simulink model "emgCalibration"  (R2017a)
settings: Solver=ode5  StartTime=0.0  StopTime=10  FixedStep=Ts_sim  RelTol=1e-3  EnableMultiTasking=on
values from neighbouring files (symbols this model uses):
  emgConst2 = 0    [initializeParameters.m]
undefined symbols (not defined in the file or in its folder): A_butter_cal, A_butter_low, B_butter_cal, B_butter_low
libraries: robotlib x1
settings Model: Creator=Clark  LastModifiedBy=jacob
settings DataIOCC: LimitDataPoints=on  SaveFormat=Array
settings OptimizationCC: LifeSpan=inf
settings DebuggingCC: SFUnexpectedBacktrackingDiag=warning  SFNoUnconditionalDefaultTransitionDiag=warning  SFExecutionAtInitializationDiag=none
settings HardwareCC: ProdBitPerPointer=32  ProdBitPerSizeT=32  ProdBitPerPtrDiffT=32  ProdLargestAtomicFloat=None  ProdIntDivRoundTo=Undefined  ProdEndianess=Unspecified  ProdWordSize=32  ProdHWDeviceType=32-bit Generic
settings ModelReferenceCC: PropagateSignalLabelsOutOfModel=off
settings GRTTargetCC: TargetLangStandard=C89/C90 (ANSI)  GeneratePreprocessorConditionals=Disable all
settings ConfigComp: CovMetricSettings=dw  CovHtmlReporting=on  CovSaveCumulativeToWorkspaceVar=on  CovSaveSingleToWorkspaceVar=on  CovExternalEMLEnable=off

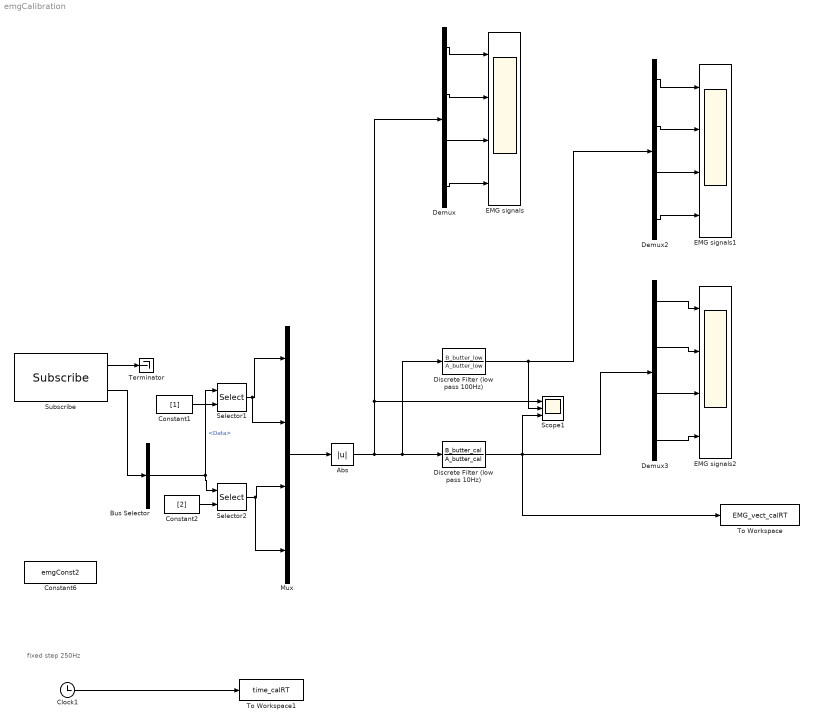
== system emgCalibration ==
  note: fixed step 250Hz
  Abs : Abs
  Bus Selector : BusSelector  OutputSignals=Data
  Clock1 : Clock
  Constant1 : Constant  Value=[1]
  Constant2 : Constant  Value=[2]
  Constant6 : Constant  Value=emgConst2  VectorParams1D=off  OutDataTypeStr=int16
  Demux : Demux
  Demux2 : Demux
  Demux3 : Demux
  Discrete Filter (low pass 100Hz) : DiscreteFilter  Numerator=B_butter_low  Denominator=A_butter_low
  Discrete Filter (low pass 10Hz) : DiscreteFilter  Numerator=B_butter_cal  Denominator=A_butter_cal
  EMG signals : Scope  NumInputPorts=4
  EMG signals1 : Scope  NumInputPorts=4
  EMG signals2 : Scope  NumInputPorts=4
  Mux : Mux
  Scope1 : Scope  NumInputPorts=3
  Selector1 : Selector  IndexOptions=Index vector (port)  Indices=[1 3]  OutputSizes=1
  Selector2 : Selector  IndexOptions=Index vector (port)  Indices=[1 3]  OutputSizes=1
  Subscribe : robotlib/Subscribe  SourceLibraryInfo=This block requires Robotics System Toolbox  topicSource=Select from ROS network  topic=/emgPub  messageType=std_msgs/Int16MultiArray  sampleTime=-1  messageQueueLength=1
      settings: SourceProductBaseCode=RO
  Terminator : Terminator
  To Workspace : ToWorkspace  VariableName=EMG_vect_calRT  SampleTime=-1
  To Workspace1 : ToWorkspace  VariableName=time_calRT  SampleTime=-1
  wires:
  Discrete Filter (low pass 10Hz)/1 -> Scope1/3, Demux3/1, To Workspace/1
  Mux/1 -> Abs/1
  Demux/1 -> EMG signals/1
  Demux/2 -> EMG signals/2
  Demux/3 -> EMG signals/3
  Demux/4 -> EMG signals/4
  Discrete Filter (low pass 100Hz)/1 -> Scope1/2, Demux2/1
  Abs/1 -> Scope1/1, Demux/1, Discrete Filter (low pass 10Hz)/1, Discrete Filter (low pass 100Hz)/1
  Demux2/1 -> EMG signals1/1
  Demux2/2 -> EMG signals1/2
  Demux2/3 -> EMG signals1/3
  Demux2/4 -> EMG signals1/4
  Demux3/1 -> EMG signals2/1
  Demux3/2 -> EMG signals2/2
  Demux3/3 -> EMG signals2/3
  Demux3/4 -> EMG signals2/4
  Clock1/1 -> To Workspace1/1
  Constant2/1 -> Selector2/2
  Subscribe/1 -> Terminator/1
  Constant1/1 -> Selector1/2
  Bus Selector/1 -> Selector2/1, Selector1/1  "<Data>"
  Selector2/1 -> Mux/4, Mux/3
  Subscribe/2 -> Bus Selector/1
  Selector1/1 -> Mux/2, Mux/1
